simulink model "untitled"  (R2017a)
settings: Solver=ode4  StartTime=0.0  StopTime=10.0  FixedStep=0.1  RelTol=1e-3
undefined symbols (not defined in the file): a, b, c, d
libraries: simulink x1
settings Model: Creator=22132  LastModifiedBy=22132

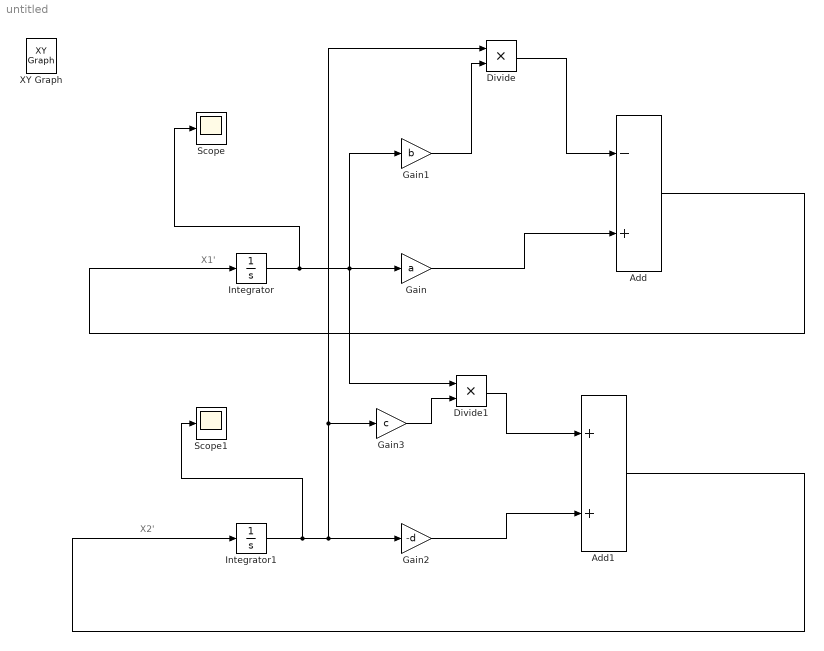
== system untitled ==
  note: X2'
  note: X1'
  Add : Sum  Inputs=-+
  Add1 : Sum
  Divide : Product  Inputs=**
  Divide1 : Product  Inputs=**
  Gain : Gain  Gain=a
  Gain1 : Gain  Gain=b
  Gain2 : Gain  Gain=-d
  Gain3 : Gain  Gain=c
  Integrator : Integrator  InitialCondition=1
  Integrator1 : Integrator
  Scope : Scope
  Scope1 : Scope
  XY Graph : simulink/Sinks/XY Graph  xmin=0  xmax=0  ymin=0  ymax=1  st=0
  wires:
  Integrator/1 -> Scope/1, Divide1/1, Gain1/1, Gain/1
  Gain/1 -> Add/2
  Integrator1/1 -> Scope1/1, Divide/1, Gain3/1, Gain2/1
  Gain1/1 -> Divide/2
  Divide/1 -> Add/1
  Add/1 -> Integrator/1
  Gain3/1 -> Divide1/2
  Divide1/1 -> Add1/1
  Gain2/1 -> Add1/2
  Add1/1 -> Integrator1/1
